simulink model "AM1"  (Simulink 8.4)
settings: Solver=ode45  StartTime=0.0  StopTime=0.5  RelTol=1e-3
undefined symbols (not defined in the file or in its folder): get
libraries: dspspect3 x1, dspsnks4 x1
settings Model: Creator=fapojuwo  LastModifiedBy=benjaminhilborn
settings DataIOCC: SignalLoggingName=sigsOut
settings DebuggingCC: SaveWithParameterizedLinksMsg=none  SignalResolutionControl=TryResolveAllWithWarning  SolverPrmCheckMsg=none  MultiTaskDSMMsg=warning  MultiTaskCondExecSysMsg=none
settings HardwareCC: TargetUnknown=on
settings RTWCC: IncludeERTFirstTime=on

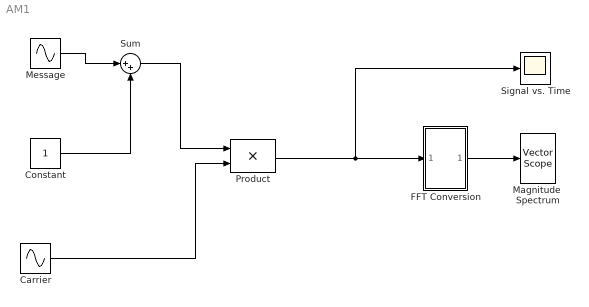
== system AM1 ==
  Carrier : Sin  Frequency=3000*2*pi  SampleTime=1/16000
      settings: AttributesFormatString=Amplitude = %<Amplitude>\nFrequency = %<Frequency>
  Constant : Constant
  FFT Conversion : Subsystem
  Magnitude  Spectrum : dspsnks4/Vector Scope  ScopeProperties=off  Domain=Frequency  HorizSpan=1  DisplayProperties=off  AxisGrid=on  Memory=off  FrameNumber=on  AxisLegend=off  AxisZoom=off  OpenScopeAtSimStart=on  OpenScopeImmediately=off  FigPos=get(0,'defaultfigureposition')  AxisProperties=on  XUnits=Hertz  XRange=[0...Fs/2]  InheritXIncr=on  XIncr=1  XLabel=Time  XLimit=Auto  XMin=0  XMax=1  XStart=0  YUnits=Magnitude  YLabel=Amplitude  LineProperties=off  XAxisParamsVer=6.8
      settings: YMin=0.000318299870930715  YMax=0.548504340064008
  Message : Sin  Amplitude=0.8  Frequency=300*2*pi  SampleTime=1/16000
      settings: AttributesFormatString=Mod. Index = %<Amplitude>\nFreq = %<Frequency>
  Product : Product  SaturateOnIntegerOverflow=on  OutDataTypeStr=Inherit: Same as first input
  Signal vs. Time : Scope
      settings: TickLabels=on  SampleInput=on  SampleTime=1/16000
  Sum : Sum  Inputs=|++  SaturateOnIntegerOverflow=on
  wires:
  Carrier/1 -> Product/2
  Message/1 -> Sum/1
  Constant/1 -> Sum/2
  Sum/1 -> Product/1
  FFT Conversion/1(Out1) -> Magnitude  Spectrum/1
  Product/1 -> FFT Conversion/1(In1), Signal vs. Time/1

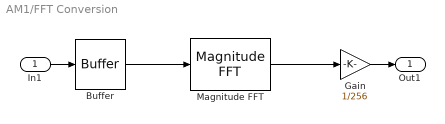
== system AM1/FFT Conversion ==
  In1 : Inport
  Buffer : Buffer  N=256
  Gain : Gain  Gain=1/256  SaturateOnIntegerOverflow=on  OutDataTypeStr=Inherit: Same as input  ParamDataTypeStr=Inherit: Same as input
  Magnitude FFT : dspspect3/Magnitude FFT  mag_or_magsq=Magnitude  FFTImplementation=Auto  fftLenInherit=off  fftsize=256  WrapInput=on
  Out1 : Outport
  wires:
  Buffer/1 -> Magnitude FFT/1
  Magnitude FFT/1 -> Gain/1
  In1/1 -> Buffer/1
  Gain/1 -> Out1/1
